simulink model "rtwdemo_clibsup"  (Simulink 7.6)
settings: Solver=FixedStepDiscrete  StartTime=0.0  StopTime=10.0  FixedStep=1  RelTol=1e-3
undefined symbols (not defined in the file or in its folder): magnitude, Newton, Raphson
libraries: rtwdemowidgets x3
Description:
  | ANSI(R) C, ISO(R) C, GNU(R) C, and ISO(R) C++ Math Library Support
settings Model: Creator=The MathWorks Inc.  ExtModeAutoUpdateStatusClock=off
settings MATStruct: SampleTime=1  Offset=0  Priority=[20.0]
settings DataIOCC: SaveOutput=off  SaveTime=off  SignalLoggingName=sigsOut
settings OptimizationCC: InlineParams=on  UseIntDivNetSlope=on  InlineInvariantSignals=on  EnhancedBackFolding=on  StateBitsets=on  DataBitsets=on  UseTempVars=on  EfficientFloat2IntCast=on
settings DebuggingCC: CheckExecutionContextPreStartOutputMsg=on  CheckExecutionContextRuntimeOutputMsg=on  SolverPrmCheckMsg=none  StrictBusMsg=ErrorOnBusTreatedAsVector
settings HardwareCC: ProdBitPerLong=64  ProdIntDivRoundTo=Zero  ProdEndianess=LittleEndian  ProdWordSize=64  ProdHWDeviceType=Specified  TargetHWDeviceType=Generic->32-bit Embedded Processor
settings RTWCC: TLCOptions=-p0 -aWarnNonSaturatedBlocks=0  GenCodeOnly=on  GenerateReport=on  RTWVerbose=off  ProcessScript=grt_make_rtw_hook  LaunchReport=on
settings CodeAppCC: ForceParamTrailComments=on

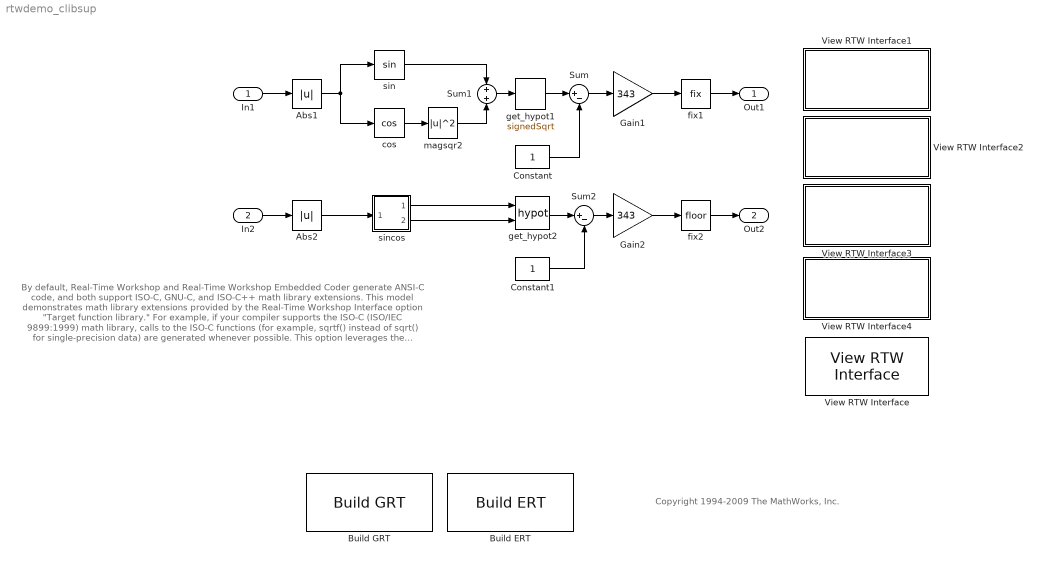
== system rtwdemo_clibsup ==
  note: By default, Real-Time Workshop and Real-Time Workshop Embedded Coder generate
      | ANSI-C code, and both support ISO-C, GNU-C, and ISO-C++ math library extensions.
      | This model demonstrates math library extensions provided by the Real-Time Workshop
      | Interface option "Target function library."
      |
      | For example, if your compiler supports the ISO-C (ISO/IEC 9899:1999) math library,
      | calls to the ISO-C functions (for example, sqrtf() instead of sqrt() for single-precision
      | data) are generated whenever possible.  This option leverages the performance your
      | target compiler offers over standard ANSI-C.
  note: Copyright 1994-2009 The MathWorks, Inc.
  In1 : Inport  OutDataTypeStr=single  PortDimensions=1  SampleTime=1
  In2 : Inport  Port=2  OutDataTypeStr=single  PortDimensions=1  SampleTime=1
  Abs1 : Abs  SaturateOnIntegerOverflow=on
  Abs2 : Abs  SaturateOnIntegerOverflow=on
  Build ERT : rtwdemowidgets/Build ERT  SystemSampleTime=-1  attrib_overrides={'GenFloatMathFcnCalls'}
  Build GRT : rtwdemowidgets/Build GRT  SystemSampleTime=-1  attrib_overrides={'GenFloatMathFcnCalls'}
  Constant : Constant  OutDataTypeStr=Inherit: Inherit via back propagation
  Constant1 : Constant  OutDataTypeStr=Inherit: Inherit via back propagation
  Gain1 : Gain  Gain=343  SaturateOnIntegerOverflow=on  OutDataTypeStr=Inherit: Same as input  ParamDataTypeStr=Inherit: Same as input
  Gain2 : Gain  Gain=343  SaturateOnIntegerOverflow=on  OutDataTypeStr=Inherit: Same as input  ParamDataTypeStr=Inherit: Same as input
  Sum : Sum  Inputs=|+-  SaturateOnIntegerOverflow=on  InputSameDT=on  OutDataTypeStr=Inherit: Same as first input
  Sum1 : Sum  SaturateOnIntegerOverflow=on  InputSameDT=on  OutDataTypeStr=Inherit: Same as first input
  Sum2 : Sum  Inputs=|+-  SaturateOnIntegerOverflow=on  InputSameDT=on  OutDataTypeStr=Inherit: Same as first input
  View RTW Interface : rtwdemowidgets/View RTW Interface  SystemSampleTime=-1
  View RTW Interface1 : Subsystem
      settings: OpenFcn=|
      | set_param(bdroot,'TargetLang','C');
      | set_param(bdroot, 'GenFloatMathFcnCalls', 'ANSI_C');
      | dlg = get_param(bdroot, 'SimPrmDialog');
      | if isa(dlg, 'DAStudio.Dialog')
      |             dlg.refresh;
      | end; clear dlg;
      mask Display: disp('Use ANSI-C (C89/C90)\nMath Library \n(double-click)')
  View RTW Interface2 : Subsystem
      settings: OpenFcn=|
      | set_param(bdroot,'TargetLang','C');
      | set_param(bdroot, 'GenFloatMathFcnCalls', 'ISO_C');
      | dlg = get_param(bdroot, 'SimPrmDialog');
      | if isa(dlg, 'DAStudio.Dialog')
      |             dlg.refresh;
      | end; clear dlg;
      mask Display: disp('Use ISO-C (C99)\nMath Library \n(double-click)')
  View RTW Interface3 : Subsystem
      settings: OpenFcn=|
      | set_param(bdroot,'TargetLang','C');
      | set_param(bdroot, 'GenFloatMathFcnCalls', 'GNU');                                                            dlg = get_param(bdroot, 'SimPrmDialog');
      | if isa(dlg, 'DAStudio.Dialog')
      |             dlg.refresh;
      | end; clear dlg;
      mask Display: disp('Use GNU-C\nMath Library \n(double-click)')
  View RTW Interface4 : Subsystem
      settings: OpenFcn=|
      | set_param(bdroot, 'TargetLang', 'C++');
      | set_param(bdroot, 'GenFloatMathFcnCalls', 'C++ (ISO)');
      | dlg = get_param(bdroot, 'SimPrmDialog');
      | if isa(dlg, 'DAStudio.Dialog')
      |             dlg.refresh;
      | end; clear dlg;
      mask Display: disp('Use ISO-C++\nMath Library \n(double-click)')
  cos : Trigonometry  Operator=cos
  fix1 : Rounding  Operator=fix
  fix2 : Rounding
  get_hypot1 : Sqrt  Operator=signedSqrt  AlgorithmType=Newton-Raphson  SaturateOnIntegerOverflow=on
  get_hypot2 : Math  Operator=hypot  SaturateOnIntegerOverflow=on
  magsqr2 : Math  Operator=magnitude^2  SaturateOnIntegerOverflow=on
  sin : Trigonometry
  sincos : Subsystem
      mask Display: text(0.5,0.5,'sincos','horizontalAlignment','center')
  Out1 : Outport
  Out2 : Outport  Port=2
  wires:
  In1/1 -> Abs1/1
  sin/1 -> Sum1/1
  cos/1 -> magsqr2/1
  get_hypot1/1 -> Sum/1
  Abs1/1 -> sin/1, cos/1
  Constant/1 -> Sum/2
  Sum/1 -> Gain1/1
  Sum1/1 -> get_hypot1/1
  magsqr2/1 -> Sum1/2
  sincos/1(Out1) -> get_hypot2/1
  sincos/2(Out2) -> get_hypot2/2
  get_hypot2/1 -> Sum2/1
  Sum2/1 -> Gain2/1
  Constant1/1 -> Sum2/2
  In2/1 -> Abs2/1
  Abs2/1 -> sincos/1(In1)
  Gain1/1 -> fix1/1
  Gain2/1 -> fix2/1
  fix1/1 -> Out1/1
  fix2/1 -> Out2/1

== system rtwdemo_clibsup/View RTW Interface1 ==

== system rtwdemo_clibsup/View RTW Interface2 ==

== system rtwdemo_clibsup/View RTW Interface3 ==

== system rtwdemo_clibsup/View RTW Interface4 ==

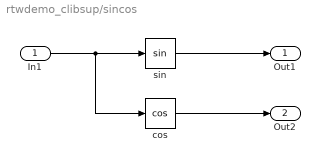
== system rtwdemo_clibsup/sincos ==
  In1 : Inport
  cos : Trigonometry  Operator=cos
  sin : Trigonometry
  Out1 : Outport
  Out2 : Outport  Port=2
  wires:
  In1/1 -> sin/1, cos/1
  sin/1 -> Out1/1
  cos/1 -> Out2/1
